simulink model "Home_5_4G"  (R2018a)
settings: Solver=VariableStepAuto  StartTime=0.0  StopTime=runtime  RelTol=1e-3
values from neighbouring files (symbols this model uses):
  Imax = 122.5    [Home54_init.m]
  J = 0.05    [Ex5_2_init.m]    (also in Ex5_3_init.m; Home54_init.m = 0.5; homepart51.m)
  Ki_w = 24000    [Home54_init.m]
  Kp_w = 320    [Home54_init.m]
  L0 = 1e-4    (= 0.0001)    [Home54_init.m]
  L_s = 0.085    [Ex5_2_init.m]    (also in Ex5_3_init.m; Home54_init.m)
  p = 1    [Ex5_2_init.m]    (also in Ex5_3_init.m; Home54_init.m; homepart51.m)
  R_R_m = R_R    (= 0.2792)    [Home54_init.m]
  rho0 = 1e-4    (= 0.0001)    [Home54_init.m]
  sigma = 1 - M^2/(L_s*L_r)    (= 0.0693425605536)    [Ex5_2_init.m]    (also in Ex5_3_init.m = 0.0693; Home54_init.m = 0.0693; homepart51.m)
  tau_r = 0.283    [Ex5_3_init.m]    (also in Home54_init.m)
  tau_r_m = tau_r    (= 0.283)    [Home54_init.m]
  Wm0 = 0    [Home54_init.m]
undefined symbols (not defined in the file or in its folder): sigbuilder_block
settings Model: Creator=Niels  LastModifiedBy=Niels
settings CodeAppCC: StateflowObjectComments=on

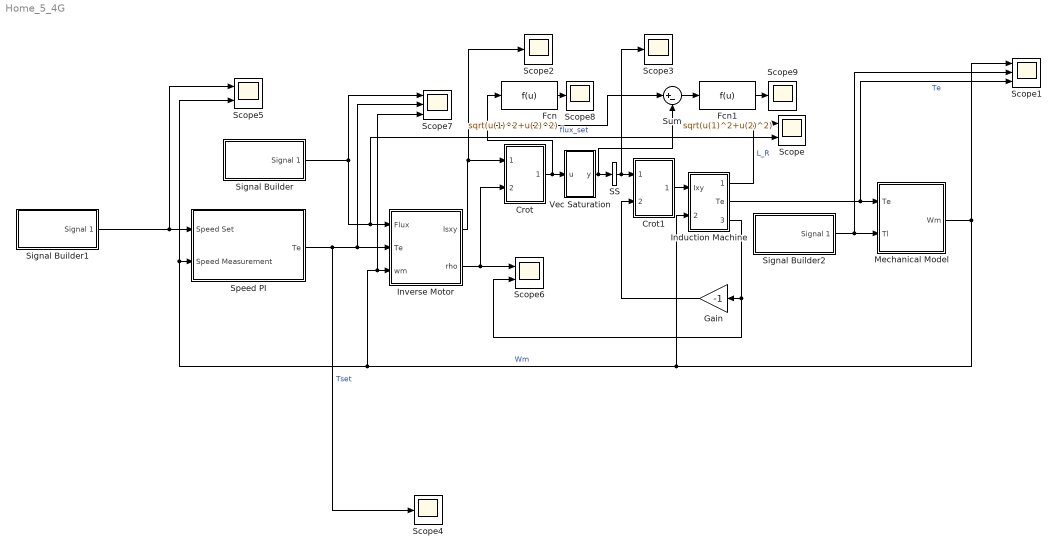
== system Home_5_4G ==
  Crot : Subsystem
  Crot1 : Subsystem
  Fcn : Fcn  Expr=sqrt(u(1)^2+u(2)^2)
  Fcn1 : Fcn  Expr=sqrt(u(1)^2+u(2)^2)
  Gain : Gain  Gain=-1
  Induction Machine : Subsystem
  Inverse Motor : Subsystem
  Mechanical Model : Subsystem
  SS : SignalSpecification  Dimensions=[2 1]
  Scope : Scope  NumInputPorts=2
  Scope1 : Scope  NumInputPorts=3
  Scope{2..4,8..9} (5 alike) : Scope
  Scope5 : Scope  NumInputPorts=2
  Scope6 : Scope  NumInputPorts=2
  Scope7 : Scope  NumInputPorts=3
  Signal Builder : Subsystem  Tag=STV Subsys  LoadFcn=sigbuilder_block('load');  StartFcn=sigbuilder_block('start');  StopFcn=sigbuilder_block('stop');  ClipboardFcn=sigbuilder_block('clipboard');  mask(Sigbuilder block){tuvar=[0:10]}
      mask help: Simulink:masks:SigbuilderBlock_MD
      mask init:
      | if ~strcmp(get_param(bdroot(gcbh),'SimulationStatus'),'stopped') tuvar = sigbuilder_block('maskInit'); end
      settings: CopyFcn=sigbuilder_block('copy');  DeleteFcn=sigbuilder_block('delete');  ModelCloseFcn=sigbuilder_block('modelClose');  PreSaveFcn=sigbuilder_block('preSave');  PauseFcn=sigbuilder_block('pause');  ContinueFcn=sigbuilder_block('continue');  NameChangeFcn=sigbuilder_block('namechange');  OpenFcn=sigbuilder_block('open',[0.75 30.75 718.5 715.5 ]);  CloseFcn=sigbuilder_block('close');
      mask Display: plot(0, 0, 100, 100,[2, 2, 32, 32, 2], [68, 8, 8, 68, 68],[32, 2], [38, 38], [32, 19, 2],[53, 60, 44], [32, 17, 17, 2],[16, 16, 31, 31]);txt = getActiveGroup(gcbh);text(2, 100, txt,'verticalAlignment', 'top');
  Signal Builder1 : Subsystem  Tag=STV Subsys  LoadFcn=sigbuilder_block('load');  StartFcn=sigbuilder_block('start');  StopFcn=sigbuilder_block('stop');  ClipboardFcn=sigbuilder_block('clipboard');  mask(Sigbuilder block){tuvar=[0:10]}
      mask help: Simulink:masks:SigbuilderBlock_MD
      mask init:
      | if ~strcmp(get_param(bdroot(gcbh),'SimulationStatus'),'stopped') tuvar = sigbuilder_block('maskInit'); end
      settings: CopyFcn=sigbuilder_block('copy');  DeleteFcn=sigbuilder_block('delete');  ModelCloseFcn=sigbuilder_block('modelClose');  PreSaveFcn=sigbuilder_block('preSave');  PauseFcn=sigbuilder_block('pause');  ContinueFcn=sigbuilder_block('continue');  NameChangeFcn=sigbuilder_block('namechange');  OpenFcn=sigbuilder_block('open',[437.6 199.2 550.4 400 ]);  CloseFcn=sigbuilder_block('close');
      mask Display: plot(0, 0, 100, 100,[2, 2, 32, 32, 2], [68, 8, 8, 68, 68],[32, 2], [38, 38], [32, 19, 2],[53, 60, 44], [32, 17, 17, 2],[16, 16, 31, 31]);txt = getActiveGroup(gcbh);text(2, 100, txt,'verticalAlignment', 'top');
  Signal Builder2 : Subsystem  Tag=STV Subsys  LoadFcn=sigbuilder_block('load');  StartFcn=sigbuilder_block('start');  StopFcn=sigbuilder_block('stop');  ClipboardFcn=sigbuilder_block('clipboard');  mask(Sigbuilder block){tuvar=[0:10]}
      mask help: Simulink:masks:SigbuilderBlock_MD
      mask init:
      | if ~strcmp(get_param(bdroot(gcbh),'SimulationStatus'),'stopped') tuvar = sigbuilder_block('maskInit'); end
      settings: CopyFcn=sigbuilder_block('copy');  DeleteFcn=sigbuilder_block('delete');  ModelCloseFcn=sigbuilder_block('modelClose');  PreSaveFcn=sigbuilder_block('preSave');  PauseFcn=sigbuilder_block('pause');  ContinueFcn=sigbuilder_block('continue');  NameChangeFcn=sigbuilder_block('namechange');  OpenFcn=sigbuilder_block('open',[437.6 199.2 550.4 400 ]);  CloseFcn=sigbuilder_block('close');
      mask Display: plot(0, 0, 100, 100,[2, 2, 32, 32, 2], [68, 8, 8, 68, 68],[32, 2], [38, 38], [32, 19, 2],[53, 60, 44], [32, 17, 17, 2],[16, 16, 31, 31]);txt = getActiveGroup(gcbh);text(2, 100, txt,'verticalAlignment', 'top');
  Speed PI : Subsystem
  Sum : Sum  Inputs=|+-
  Vec Saturation : MATLAB Function  TreatAsAtomicUnit=on
  wires:
  Mechanical Model/1(Wm) -> Scope1/1, Scope7/3, Inverse Motor/3(wm), Scope5/2, Speed PI/2(Speed Measurement), Induction Machine/2(Wm)  "Wm"
  Induction Machine/2(Te) -> Scope1/3, Mechanical Model/1(Te)  "Te"
  Signal Builder2/1(Signal 1) -> Scope1/2, Mechanical Model/2(Tl)
  Induction Machine/3(rho) -> Scope6/2, Gain/1
  Crot/1(Ialpbet) -> Sum/1, Fcn/1, Vec Saturation/1(u)
  Crot1/1(Isxy) -> Induction Machine/1(Ixy)
  Gain/1 -> Crot1/2(-rho)
  Vec Saturation/1(y) -> Sum/2, SS/1
  SS/1 -> Scope3/1, Crot1/1(Ialphbet)
  Speed PI/1(Te) -> Scope4/1, Scope7/2, Inverse Motor/2(Te)  "Tset"
  Inverse Motor/1("Isxy ") -> Scope2/1, Crot/1(Isxy)
  Inverse Motor/2(rho) -> Scope6/1, Crot/2(rho)
  Induction Machine/1(L_R) -> Scope/1  "L_R"
  Signal Builder1/1(Signal 1) -> Scope5/1, Speed PI/1(Speed Set)
  Signal Builder/1(Signal 1) -> Scope7/1, Scope/2, Inverse Motor/1(Flux)  "flux_set"
  Fcn/1 -> Scope8/1
  Sum/1 -> Fcn1/1
  Fcn1/1 -> Scope9/1

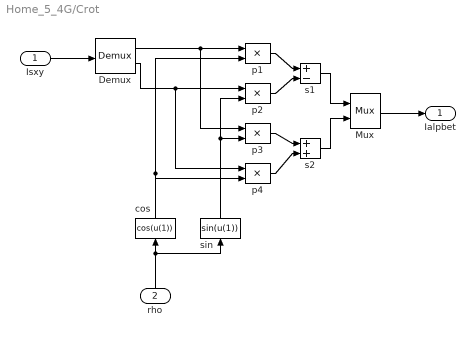
== system Home_5_4G/Crot ==
  Isxy : Inport
  rho : Inport  Port=2
  Demux : Demux  Outputs=2
  Mux : Mux  Inputs=2
  cos : Fcn  Expr=cos(u(1))
  p{1..4} (4 alike) : Product  SaturateOnIntegerOverflow=on  RndMeth=Zero  InputSameDT=on  OutDataTypeStr=Inherit: Same as first input
  s1 : Sum  Inputs=+-  SaturateOnIntegerOverflow=on  InputSameDT=on  OutDataTypeStr=Inherit: Same as first input
  s2 : Sum  SaturateOnIntegerOverflow=on  InputSameDT=on  OutDataTypeStr=Inherit: Same as first input
  sin : Fcn  Expr=sin(u(1))
  Ialpbet : Outport
  wires:
  sin/1 -> p2/2, p3/2
  cos/1 -> p1/2, p4/2
  rho/1 -> cos/1, sin/1
  Isxy/1 -> Demux/1
  p2/1 -> s1/2
  s1/1 -> Mux/1
  Demux/1 -> p1/1, p3/1
  Mux/1 -> Ialpbet/1
  Demux/2 -> p2/1, p4/1
  s2/1 -> Mux/2
  p3/1 -> s2/1
  p1/1 -> s1/1
  p4/1 -> s2/2

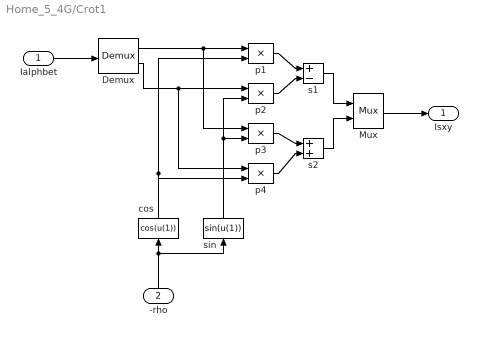
== system Home_5_4G/Crot1 ==
  Ialphbet : Inport
  -rho : Inport  Port=2
  Demux : Demux  Outputs=2
  Mux : Mux  Inputs=2
  cos : Fcn  Expr=cos(u(1))
  p{1..4} (4 alike) : Product  SaturateOnIntegerOverflow=on  RndMeth=Zero  InputSameDT=on  OutDataTypeStr=Inherit: Same as first input
  s1 : Sum  Inputs=+-  SaturateOnIntegerOverflow=on  InputSameDT=on  OutDataTypeStr=Inherit: Same as first input
  s2 : Sum  SaturateOnIntegerOverflow=on  InputSameDT=on  OutDataTypeStr=Inherit: Same as first input
  sin : Fcn  Expr=sin(u(1))
  Isxy : Outport
  wires:
  sin/1 -> p2/2, p3/2
  cos/1 -> p1/2, p4/2
  -rho/1 -> cos/1, sin/1
  Ialphbet/1 -> Demux/1
  p2/1 -> s1/2
  s1/1 -> Mux/1
  Demux/1 -> p1/1, p3/1
  Mux/1 -> Isxy/1
  Demux/2 -> p2/1, p4/1
  s2/1 -> Mux/2
  p3/1 -> s2/1
  p1/1 -> s1/1
  p4/1 -> s2/2

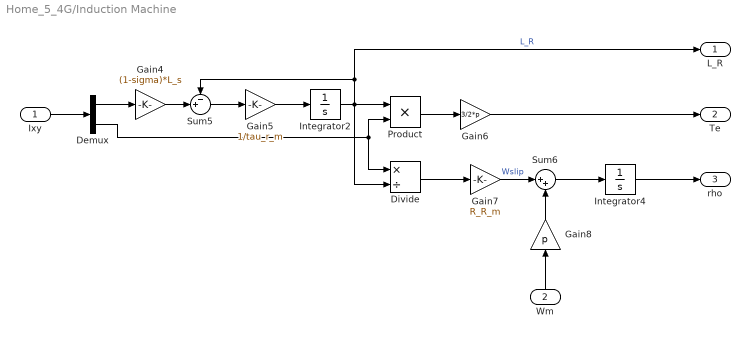
== system Home_5_4G/Induction Machine ==
  Ixy : Inport
  Wm : Inport  Port=2
  Demux : Demux  Outputs=2
  Divide : Product  Inputs=*/
  Gain4 : Gain  Gain=(1-sigma)*L_s
  Gain5 : Gain  Gain=1/tau_r_m
  Gain6 : Gain  Gain=3/2*p
  Gain7 : Gain  Gain=R_R_m
  Gain8 : Gain  Gain=p
  Integrator2 : Integrator  InitialCondition=L0
  Integrator4 : Integrator  InitialCondition=rho0
  Product : Product
  Sum5 : Sum  Inputs=-+|
  Sum6 : Sum  Inputs=|++
  L_R : Outport
  Te : Outport  Port=2
  rho : Outport  Port=3
  wires:
  Gain5/1 -> Integrator2/1
  Gain4/1 -> Sum5/2
  Sum6/1 -> Integrator4/1
  Sum5/1 -> Gain5/1
  Demux/2 -> Divide/1, Product/2
  Gain6/1 -> Te/1
  Demux/1 -> Gain4/1
  Ixy/1 -> Demux/1
  Integrator2/1 -> Divide/2, Product/1, L_R/1, Sum5/1  "L_R"
  Divide/1 -> Gain7/1
  Gain8/1 -> Sum6/2
  Wm/1 -> Gain8/1
  Gain7/1 -> Sum6/1  "Wslip"
  Product/1 -> Gain6/1
  Integrator4/1 -> rho/1

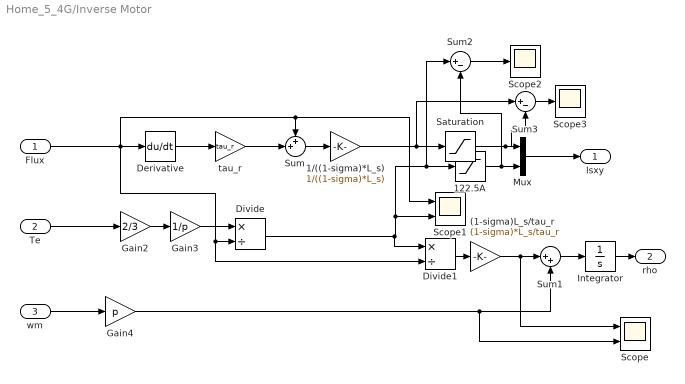
== system Home_5_4G/Inverse Motor ==
  Flux : Inport
  Te : Inport  Port=2
  wm : Inport  Port=3
  (1-sigma)L_s/tau_r : Gain  Gain=(1-sigma)*L_s/tau_r
  1/((1-sigma)*L_s) : Gain  Gain=1/((1-sigma)*L_s)
  122.5A : Saturate  UpperLimit=Imax  LowerLimit=-Imax
  Derivative : Derivative
  Divide : Product  Inputs=*/
  Divide1 : Product  Inputs=*/
  Gain2 : Gain  Gain=2/3
  Gain3 : Gain  Gain=1/p
  Gain4 : Gain  Gain=p
  Integrator : Integrator
  Mux : Mux  Inputs=2
  Saturation : Saturate  UpperLimit=Imax  LowerLimit=-Imax
  Scope : Scope  NumInputPorts=2
  Scope1 : Scope  NumInputPorts=2
  Scope2 : Scope
  Scope3 : Scope
  Sum : Sum  Inputs=++|
  Sum1 : Sum  Inputs=|++
  Sum2 : Sum  Inputs=|+-
  Sum3 : Sum  Inputs=|+-
  tau_r : Gain  Gain=tau_r
  "Isxy " : Outport
  rho : Outport  Port=2
  wires:
  Derivative/1 -> tau_r/1
  tau_r/1 -> Sum/2
  Sum/1 -> 1/((1-sigma)*L_s)/1
  1/((1-sigma)*L_s)/1 -> Sum3/1, Saturation/1
  Te/1 -> Gain2/1
  Gain2/1 -> Gain3/1
  Gain3/1 -> Divide/1
  Divide/1 -> Divide1/1, Scope1/2, Sum2/1, 122.5A/1
  wm/1 -> Gain4/1
  Mux/1 -> "Isxy "/1
  Flux/1 -> Divide1/2, Divide/2, Scope1/1, Sum/1, Derivative/1
  Gain4/1 -> Scope/2, Sum1/2
  Sum1/1 -> Integrator/1
  Integrator/1 -> rho/1
  Saturation/1 -> Sum3/2, Mux/1
  122.5A/1 -> Sum2/2, Mux/2
  (1-sigma)L_s/tau_r/1 -> Scope/1, Sum1/1
  Divide1/1 -> (1-sigma)L_s/tau_r/1
  Sum2/1 -> Scope2/1
  Sum3/1 -> Scope3/1

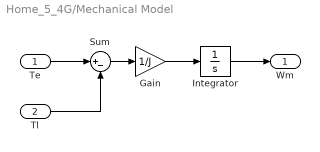
== system Home_5_4G/Mechanical Model ==
  Te : Inport
  Tl : Inport  Port=2
  Gain : Gain  Gain=1/J
  Integrator : Integrator  InitialCondition=Wm0
  Sum : Sum  Inputs=|+-
  Wm : Outport
  wires:
  Te/1 -> Sum/1
  Tl/1 -> Sum/2
  Gain/1 -> Integrator/1
  Sum/1 -> Gain/1
  Integrator/1 -> Wm/1

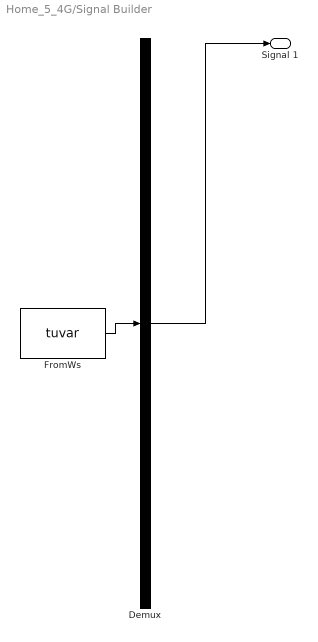
== system Home_5_4G/Signal Builder ==
  Demux : Demux  Tag=STV Demux  Outputs=1
  FromWs : FromWorkspace  Tag=STV FromWs  VariableName=tuvar  SampleTime=0
      SigBuilderData=|
      | common.afterFinalStr = 'Extrapolate'
      | common.sampleTime = 0
      | dataSet.timeRange = [0 10]
      | dataSet.name = 'Group 1'
      | sbobj.Groups.Name = 'Group 1'
      | sbobj.Groups.Signals.Name = 'Signal 1'
      | sbobj.Groups.Signals.XData = [0 0.01 0.0365 10]
      | sbobj.Groups.Signals.YData = [0.001 0.001 0.816 0.816]
  Signal 1 : Outport  Tag=STV Outport
  wires:
  Demux/1 -> Signal 1/1
  FromWs/1 -> Demux/1

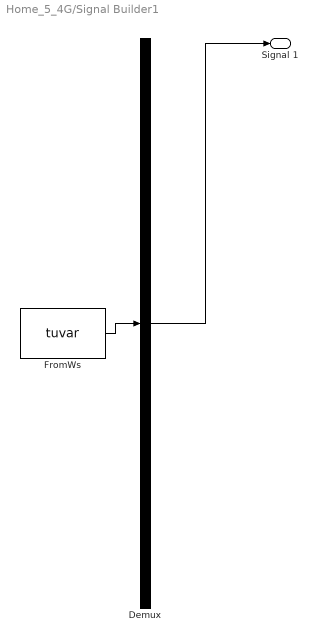
== system Home_5_4G/Signal Builder1 ==
  Demux : Demux  Tag=STV Demux  Outputs=1
  FromWs : FromWorkspace  Tag=STV FromWs  VariableName=tuvar  SampleTime=0
      SigBuilderData=|
      | common.afterFinalStr = 'Extrapolate'
      | common.sampleTime = 0
      | dataSet.timeRange = [0 50]
      | dataSet.name = 'Group 1'
      | sbobj.Groups.Name = 'Group 1'
      | sbobj.Groups.Signals.Name = 'Signal 1'
      | sbobj.Groups.Signals.XData = [0 0.1 0.1 50]
      | sbobj.Groups.Signals.YData = [0 0 300 300]
      | sbobj.Groups.TimeRange = [0 50]
  Signal 1 : Outport  Tag=STV Outport
  wires:
  Demux/1 -> Signal 1/1
  FromWs/1 -> Demux/1

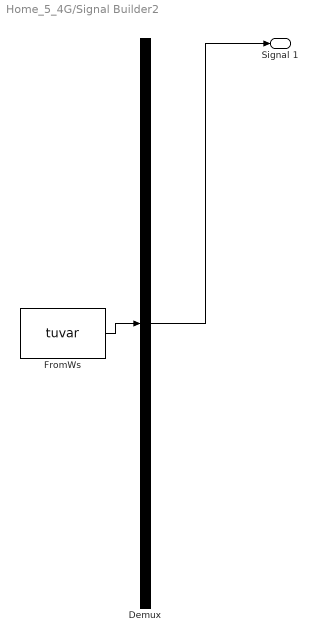
== system Home_5_4G/Signal Builder2 ==
  Demux : Demux  Tag=STV Demux  Outputs=1
  FromWs : FromWorkspace  Tag=STV FromWs  VariableName=tuvar  SampleTime=0
      SigBuilderData=|
      | common.afterFinalStr = 'Extrapolate'
      | common.sampleTime = 0
      | dataSet.timeRange = [0 50]
      | dataSet.name = 'Group 1'
      | sbobj.Groups.Name = 'Group 1'
      | sbobj.Groups.Signals.Name = 'Signal 1'
      | sbobj.Groups.Signals.XData = [0 1.5 1.5 50]
      | sbobj.Groups.Signals.YData = [0 0 50 50]
      | sbobj.Groups.TimeRange = [0 50]
  Signal 1 : Outport  Tag=STV Outport
  wires:
  Demux/1 -> Signal 1/1
  FromWs/1 -> Demux/1

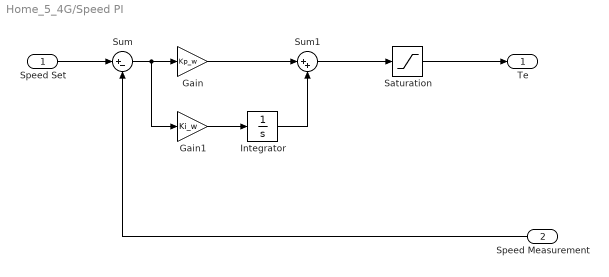
== system Home_5_4G/Speed PI ==
  Speed Set : Inport
  Speed Measurement : Inport  Port=2
  Gain : Gain  Gain=Kp_w
  Gain1 : Gain  Gain=Ki_w
  Integrator : Integrator  LimitOutput=on  UpperSaturationLimit=122.5  LowerSaturationLimit=-122.5
  Saturation : Saturate  UpperLimit=149  LowerLimit=-122.5
  Sum : Sum  Inputs=|+-
  Sum1 : Sum  Inputs=|++
  Te : Outport
  wires:
  Integrator/1 -> Sum1/2
  Speed Measurement/1 -> Sum/2
  Sum/1 -> Gain1/1, Gain/1
  Speed Set/1 -> Sum/1
  Gain1/1 -> Integrator/1
  Gain/1 -> Sum1/1
  Sum1/1 -> Saturation/1
  Saturation/1 -> Te/1

== matlab function Home_5_4G/Vec Saturation ==
  data: u input; y output; Imax parameter
function y = fcn(u,Imax)
y = u;
if u(1) >= Imax
    u(1) = Imax;
elseif u(1) <= -Imax
    u(1) = Imax;
end
if u(2) >= Imax
    u(2) = Imax;
elseif u(2) <= -Imax
    u(2) = Imax;
end
